simulink model "hardware_basic"  (R2020b)
settings: Solver=ode1  StartTime=0.0  StopTime=2000  FixedStep=0.001  RelTol=1e-3  EnableMultiTasking=on
values from neighbouring files (symbols this model uses):
  K_AMP = 3    [advanced_model_setup.m]    (also in setup_lab_hover.m; setup_physical.m; simulate_hover.m)
  K_EC_P = 2 * pi / ( 8 * 1024 )    (= 0.000766990393943)    [advanced_model_setup.m]    (also in setup_lab_hover.m; setup_physical.m; simulate_hover.m)
  K_EC_R = 2 * pi / ( 8 * 1024 )    (= 0.000766990393943)    [advanced_model_setup.m]    (also in setup_lab_hover.m; setup_physical.m; simulate_hover.m)
  K_EC_Y = -2 * pi / ( 8 * 1024 )    (= -0.000766990393943)    [advanced_model_setup.m]    (also in setup_lab_hover.m; setup_physical.m; simulate_hover.m)
  VMAX_AMP = 24    [advanced_model_setup.m]    (also in setup_lab_hover.m; setup_physical.m; simulate_hover.m)
  wcf = 2 * pi * 20    (= 125.663706144)    [advanced_model_setup.m]    (also in setup_lab_hover.m; setup_physical.m; simulate_hover.m = 628.318530718)
  zetaf = 0.6    [advanced_model_setup.m]    (also in setup_lab_hover.m; setup_physical.m; simulate_hover.m)
undefined symbols (not defined in the file or in its folder): HIL, qc_get_step_size
libraries: quarc_library x3, simulink_extras x1
settings Model: SimulationMode=external  ExtModeTrigDuration=10000  Creator=hpineros  LastModifiedBy=256444
settings SolverCC: PositivePriorityOrder=on
settings DataIOCC: MaxDataPoints=5000  SaveFormat=Array  SignalLoggingSaveFormat=ModelDataLogs  InspectSignalLogs=on  ReturnWorkspaceOutputs=off
settings OptimizationCC: ExpressionDepthLimit=2147483647  InitFltsAndDblsToZero=on  LifeSpan=inf
settings DebuggingCC: SaveWithParameterizedLinksMsg=none  UnderspecifiedInitializationDetection=Classic  MergeDetectMultiDrivingBlocksExec=none  SolverPrmCheckMsg=warning  FcnCallInpInsideContextMsg=warning  StateNameClashWarn=warning  SFUnexpectedBacktrackingDiag=warning  SFNoUnconditionalDefaultTransitionDiag=warning  SFExecutionAtInitializationDiag=none  ArithmeticOperatorsInVariantConditions=warning
settings HardwareCC: ProdBitPerPointer=32  ProdBitPerSizeT=32  ProdBitPerPtrDiffT=32  ProdLargestAtomicFloat=None  ProdIntDivRoundTo=Undefined  ProdEndianess=Unspecified  ProdWordSize=32  ProdHWDeviceType=32-bit Generic
settings ModelReferenceCC: PropagateSignalLabelsOutOfModel=off
settings SFSimCC: SimUseLocalCustomCode=off  CustomCodeUndefinedFunction=UseInterfaceOnly
settings RTWCC: Description=QUARC Win64 Target  SystemTargetFile=quarc_win64.tlc  TemplateMakefile=quarc_default_tmf  RTWUseLocalCustomCode=off
settings CodeAppCC: StateflowObjectComments=on
settings STFCustomTargetCC: CombineOutputUpdateFcns=on  GRTInterface=off
settings GRTTargetCC: TargetLangStandard=C89/C90 (ANSI)  ParMdlRefBuildCompliant=off  CompOptLevelCompliant=off  MatFileLogging=off  UseToolchainInfoCompliant=off  ExtMode=on  ExtModeMexFile=quarc_comm
settings ConfigComp: CovMetricSettings=dw  CovSaveCumulativeToWorkspaceVar=on  CovSaveSingleToWorkspaceVar=on  CovExternalEMLEnable=off

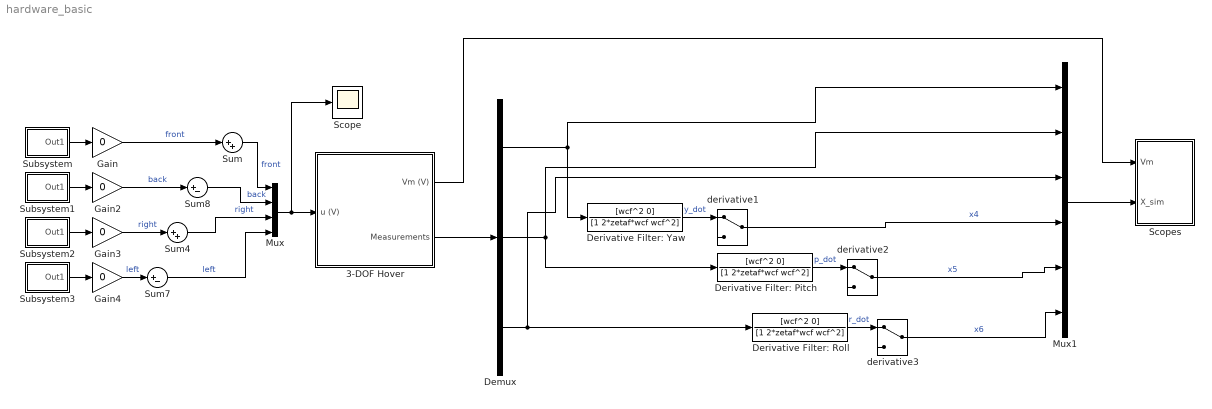
== system hardware_basic ==
  3-DOF Hover : Subsystem
  Demux : Demux  Outputs=3
  Derivative Filter: Pitch : TransferFcn  Numerator=[wcf^2 0]  Denominator=[1 2*zetaf*wcf wcf^2]
  Derivative Filter: Roll : TransferFcn  Numerator=[wcf^2 0]  Denominator=[1 2*zetaf*wcf wcf^2]
  Derivative Filter: Yaw : TransferFcn  Numerator=[wcf^2 0]  Denominator=[1 2*zetaf*wcf wcf^2]
  Gain{,2..4} (4 alike) : Gain  Gain=0
  Mux : Mux
  Mux1 : Mux  Inputs=6
  Scope : Scope
  Scopes : Subsystem
  Subsystem : Subsystem  mask{tStart=1, tStop=2, amp=1}
      mask prompts: tStart "Start time"; tStop "Stop time"; amp "Amplitude"
  Subsystem1 : Subsystem  mask{tStart=6, tStop=7, amp=1}
      mask prompts: tStart "Start time"; tStop "Stop time"; amp "Amplitude"
  Subsystem2 : Subsystem  mask{tStart=11, tStop=12, amp=1}
      mask prompts: tStart "Start time"; tStop "Stop time"; amp "Amplitude"
  Subsystem3 : Subsystem  mask{tStart=16, tStop=17, amp=1}
      mask prompts: tStart "Start time"; tStop "Stop time"; amp "Amplitude"
  Sum : Sum  Inputs=|++
  Sum4 : Sum  Inputs=|++
  Sum7 : Sum  Inputs=|+-
  Sum8 : Sum  Inputs=|+-
  derivative1 : ManualSwitch
  derivative2 : ManualSwitch
  derivative3 : ManualSwitch
  wires:
  Demux/3 -> Mux1/3, Derivative Filter: Roll/1
  Demux/1 -> Mux1/1, Derivative Filter: Yaw/1
  derivative2/1 -> Mux1/5  "x5"
  derivative1/1 -> Mux1/4  "x4"
  Demux/2 -> Mux1/2, Derivative Filter: Pitch/1
  Derivative Filter: Pitch/1 -> derivative2/1  "p_dot"
  Derivative Filter: Roll/1 -> derivative3/1  "r_dot"
  Derivative Filter: Yaw/1 -> derivative1/1  "y_dot"
  3-DOF Hover/2(Measurements) -> Demux/1
  derivative3/1 -> Mux1/6  "x6"
  Mux1/1 -> Scopes/2(X_sim)
  3-DOF Hover/1(Vm (V)) -> Scopes/1(Vm)
  Sum/1 -> Mux/1  "front"
  Sum4/1 -> Mux/3  "right"
  Sum7/1 -> Mux/4  "left"
  Subsystem1/1(Out1) -> Gain2/1
  Subsystem3/1(Out1) -> Gain4/1
  Gain4/1 -> Sum7/1  "left"
  Subsystem/1(Out1) -> Gain/1
  Subsystem2/1(Out1) -> Gain3/1
  Sum8/1 -> Mux/2  "back"
  Gain3/1 -> Sum4/1  "right"
  Mux/1 -> Scope/1, 3-DOF Hover/1(u (V))
  Gain2/1 -> Sum8/1  "back"
  Gain/1 -> Sum/1  "front"

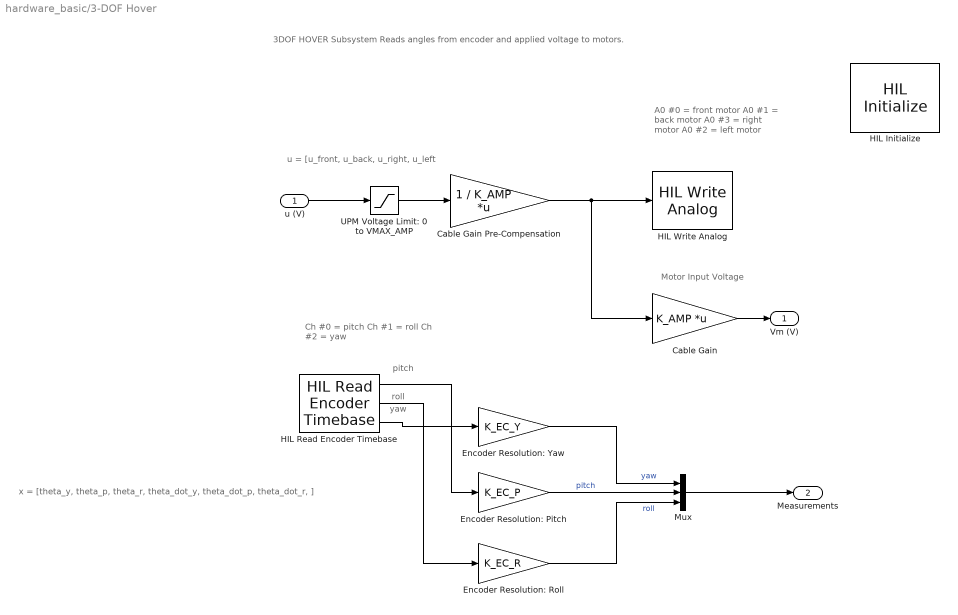
== system hardware_basic/3-DOF Hover ==
  note: roll
  note: pitch
  note: yaw
  note: Motor Input Voltage
  note: x = [theta_y, theta_p, theta_r, theta_dot_y, theta_dot_p, theta_dot_r, ]
  note: A0 #0 = front motor
      | A0 #1 = back motor
      | A0 #3 = right motor
      | A0 #2 = left motor
  note: u = [u_front, u_back, u_right, u_left
  note: 3DOF HOVER Subsystem
      | Reads angles from encoder and applied voltage to motors.
  note: Ch #0 = pitch
      | Ch #1 = roll
      | Ch #2 = yaw
  u (V) : Inport
  Cable Gain : Gain  Gain=K_AMP  Multiplication=Matrix(K*u)  SaturateOnIntegerOverflow=on  OutDataTypeStr=Inherit: Same as input  ParamDataTypeStr=Inherit: Same as input
  Cable Gain Pre-Compensation : Gain  Gain=1 / K_AMP  Multiplication=Matrix(K*u)  SaturateOnIntegerOverflow=on  OutDataTypeStr=Inherit: Same as input  ParamDataTypeStr=Inherit: Same as input
  Encoder Resolution: Pitch : Gain  Gain=K_EC_P
  "Encoder Resolution: Roll " : Gain  Gain=K_EC_R
  Encoder Resolution: Yaw : Gain  Gain=K_EC_Y
  HIL Initialize : quarc_library/Data Acquisition/Generic/Configuration/HIL Initialize  object_name=HIL-1  board_type=q8_usb  board_number=0  board_options=update_rate=normal  exclusive=off  active=on  hardware_clocks=[0:2]  clock_modes=[]  initial_clock_frequencies=[]  set_clock_params_at_start=off  set_clock_params_at_switch_in=off  set_clock_frequencies_at_start=off  set_clock_frequencies_at_switch_in=off  analog_input_channels=[0:7]  analog_input_configurations=[]  analog_input_maximums=10  analog_input_minimums=-10  set_analog_input_params_at_start=on  set_analog_input_params_at_switch_in=off  analog_output_channels=[0:7]  analog_output_maximums=10  analog_output_minimums=-10  initial_analog_outputs=[0]  final_analog_outputs=[0]  watchdog_analog_outputs=0  set_analog_output_params_at_start=on  set_analog_output_params_at_switch_in=off  set_analog_outputs_at_start=on  set_analog_outputs_at_switch_in=off  set_analog_outputs_at_terminate=on  set_analog_outputs_at_switch_out=off  set_analog_outputs_on_watchdog=off  digital_input_channels=[]  digital_output_channels=[0:3]  digital_output_configuration=[]  initial_digital_outputs=[0]  final_digital_outputs=[0]  watchdog_digital_outputs=[0]  set_digital_output_params_at_start=off  set_digital_output_params_at_switch_in=off  set_digital_outputs_at_start=on  set_digital_outputs_at_switch_in=off  set_digital_outputs_at_terminate=on  set_digital_outputs_at_switch_out=off  set_digital_outputs_on_watchdog=off  encoder_channels=[0:7]  quadrature=[4]  encoder_filter_frequency=[]  initial_encoder_counts=[0]  set_encoder_params_at_start=on  set_encoder_params_at_switch_in=off  set_encoder_counts_at_start=on  set_encoder_counts_at_switch_in=off  pwm_channels=[0:7]  pwm_modes=0  pwm_frequency=99.532799999999995e6/4095  pwm_configuration=[0]  pwm_alignment=[0]  pwm_polarity=[1]  pwm_leading_deadband=[0]  pwm_trailing_deadband=[0]  initial_pwm_outputs=[0]  final_pwm_outputs=[0]  watchdog_pwm_outputs=[0]  set_pwm_params_at_start=on  set_pwm_params_at_switch_in=off  set_pwm_outputs_at_start=on  set_pwm_outputs_at_switch_in=off  set_pwm_outputs_at_terminate=on  set_pwm_outputs_at_switch_out=off  set_pwm_outputs_on_watchdog=off  other_output_channels=[]  initial_other_outputs=[]  final_other_outputs=[]  watchdog_other_outputs=[]  set_other_outputs_at_start=off  set_other_outputs_at_switch_in=off  set_other_outputs_at_terminate=off  set_other_outputs_at_switch_out=off  set_other_outputs_on_watchdog=off
  HIL Read Encoder Timebase : quarc_library/Data Acquisition/Generic/Timebases/HIL Read Encoder Timebase  object_name=HIL-1  clock=0  channels=[0:2]  active=on  vector_output=off  data_type_mode=Inherit via back propagation  data_type=double  overflow_mode=Error on overflow  samples_in_buffer=max(ceil(1/qc_get_step_size), 1)
  HIL Write Analog : quarc_library/Data Acquisition/Generic/Immediate I//O/HIL Write Analog  object_name=HIL-1  channels=[0,1,2,3]  sample_time=-1  active=off  vector_input=on
  Mux : Mux  Inputs=3
  UPM Voltage Limit: 0 to VMAX_AMP : Saturate  UpperLimit=VMAX_AMP  LowerLimit=0
  Vm (V) : Outport
  Measurements : Outport  Port=2
  wires:
  Cable Gain Pre-Compensation/1 -> Cable Gain/1, HIL Write Analog/1
  HIL Read Encoder Timebase/3 -> Encoder Resolution: Yaw/1
  HIL Read Encoder Timebase/1 -> Encoder Resolution: Pitch/1
  HIL Read Encoder Timebase/2 -> "Encoder Resolution: Roll "/1
  UPM Voltage Limit: 0 to VMAX_AMP/1 -> Cable Gain Pre-Compensation/1
  Cable Gain/1 -> Vm (V)/1
  u (V)/1 -> UPM Voltage Limit: 0 to VMAX_AMP/1
  "Encoder Resolution: Roll "/1 -> Mux/3  "roll"
  Encoder Resolution: Yaw/1 -> Mux/1  "yaw"
  Encoder Resolution: Pitch/1 -> Mux/2  "pitch"
  Mux/1 -> Measurements/1

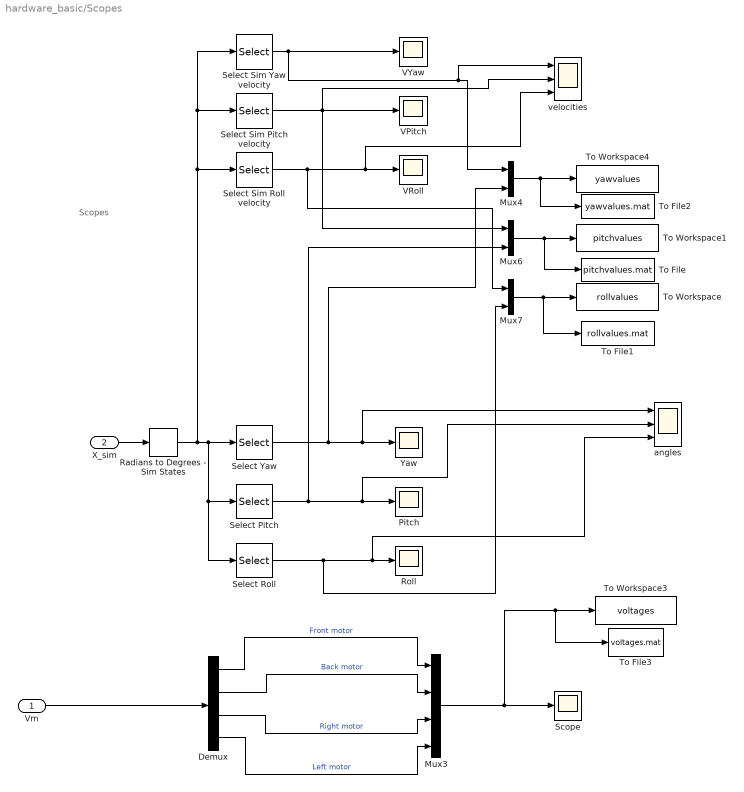
== system hardware_basic/Scopes ==
  note: Scopes
  Vm : Inport
  X_sim : Inport  Port=2
  Demux : Demux
  Mux3 : Mux
  Mux4 : Mux  Inputs=2
  Mux6 : Mux  Inputs=2
  Mux7 : Mux  Inputs=2
  Pitch : Scope
  Radians to Degrees - Sim States : simulink_extras/Transformations/Radians to Degrees
  Roll : Scope
  Scope : Scope
  Select Pitch : Selector  InputPortWidth=6  IndexOptions=Index vector (dialog)  Indices=2  OutputSizes=1
  Select Roll : Selector  InputPortWidth=6  IndexOptions=Index vector (dialog)  Indices=3  OutputSizes=1
  Select Sim Pitch velocity : Selector  InputPortWidth=6  IndexOptions=Index vector (dialog)  Indices=5  OutputSizes=1
  Select Sim Roll velocity : Selector  InputPortWidth=6  IndexOptions=Index vector (dialog)  Indices=6  OutputSizes=1
  Select Sim Yaw velocity : Selector  InputPortWidth=6  IndexOptions=Index vector (dialog)  Indices=4  OutputSizes=1
  Select Yaw : Selector  InputPortWidth=6  IndexOptions=Index vector (dialog)  Indices=1  OutputSizes=1
  To File : ToFile  Filename=pitchvalues.mat
  To File1 : ToFile  Filename=rollvalues.mat
  To File2 : ToFile  Filename=yawvalues.mat
  To File3 : ToFile  Filename=voltages.mat
  To Workspace : ToWorkspace  VariableName=rollvalues  SampleTime=-1
  To Workspace1 : ToWorkspace  VariableName=pitchvalues  SampleTime=-1
  To Workspace3 : ToWorkspace  VariableName=voltages  SampleTime=-1
  To Workspace4 : ToWorkspace  VariableName=yawvalues  SampleTime=-1
  VPitch : Scope
  VRoll : Scope
  VYaw : Scope
  Yaw : Scope
  angles : Scope  NumInputPorts=3
  velocities : Scope  NumInputPorts=3
  wires:
  Select Roll/1 -> angles/3, Roll/1, Mux7/2
  Radians to Degrees - Sim States/1 -> Select Sim Roll velocity/1, Select Sim Pitch velocity/1, Select Sim Yaw velocity/1, Select Roll/1, Select Pitch/1, Select Yaw/1
  Select Pitch/1 -> angles/2, Pitch/1, Mux6/2
  X_sim/1 -> Radians to Degrees - Sim States/1
  Demux/1 -> Mux3/1  "Front motor"
  Demux/2 -> Mux3/2  "Back motor"
  Demux/3 -> Mux3/3  "Right motor"
  Demux/4 -> Mux3/4  "Left motor"
  Vm/1 -> Demux/1
  Select Sim Yaw velocity/1 -> VYaw/1, velocities/1, Mux4/1
  Select Sim Roll velocity/1 -> velocities/3, VRoll/1, Mux7/1
  Select Sim Pitch velocity/1 -> Mux6/1, velocities/2, VPitch/1
  Mux3/1 -> To File3/1, To Workspace3/1, Scope/1
  Select Yaw/1 -> angles/1, Yaw/1, Mux4/2
  Mux7/1 -> To File1/1, To Workspace/1
  Mux6/1 -> To File/1, To Workspace1/1
  Mux4/1 -> To File2/1, To Workspace4/1

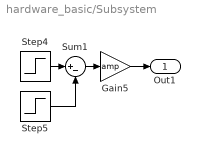
== system hardware_basic/Subsystem ==
  Gain5 : Gain  Gain=amp
  Step4 : Step  Time=tStart  SampleTime=0
  Step5 : Step  Time=tStop  SampleTime=0
  Sum1 : Sum  Inputs=|+-
  Out1 : Outport
  wires:
  Step5/1 -> Sum1/2
  Step4/1 -> Sum1/1
  Sum1/1 -> Gain5/1
  Gain5/1 -> Out1/1

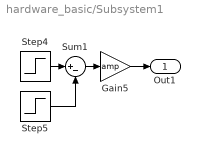
== system hardware_basic/Subsystem1 ==
  Gain5 : Gain  Gain=amp
  Step4 : Step  Time=tStart  SampleTime=0
  Step5 : Step  Time=tStop  SampleTime=0
  Sum1 : Sum  Inputs=|+-
  Out1 : Outport
  wires:
  Step5/1 -> Sum1/2
  Step4/1 -> Sum1/1
  Sum1/1 -> Gain5/1
  Gain5/1 -> Out1/1

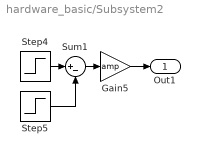
== system hardware_basic/Subsystem2 ==
  Gain5 : Gain  Gain=amp
  Step4 : Step  Time=tStart  SampleTime=0
  Step5 : Step  Time=tStop  SampleTime=0
  Sum1 : Sum  Inputs=|+-
  Out1 : Outport
  wires:
  Step5/1 -> Sum1/2
  Step4/1 -> Sum1/1
  Sum1/1 -> Gain5/1
  Gain5/1 -> Out1/1

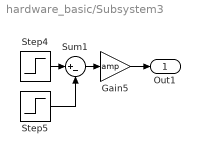
== system hardware_basic/Subsystem3 ==
  Gain5 : Gain  Gain=amp
  Step4 : Step  Time=tStart  SampleTime=0
  Step5 : Step  Time=tStop  SampleTime=0
  Sum1 : Sum  Inputs=|+-
  Out1 : Outport
  wires:
  Step5/1 -> Sum1/2
  Step4/1 -> Sum1/1
  Sum1/1 -> Gain5/1
  Gain5/1 -> Out1/1
